simulink model "AdvancedMechM34"  (R2022b)
settings: Solver=FixedStepDiscrete  StartTime=0.0  StopTime=40  FixedStep=0.01  RelTol=1e-3  EnableMultiTasking=on
undefined symbols (not defined in the file): sigbuilder_block
settings Model: SILPILSystemUnderTest=refmodels  Creator=ahmed  LastModifiedBy=Mohamed
settings SolverCC: PositivePriorityOrder=on
settings OptimizationCC: EnhancedBackFolding=on  PassReuseOutputArgsAs=Individual arguments  ZeroExternalMemoryAtStartup=off  ZeroInternalMemoryAtStartup=off  MaxStackSize=64  OptimizeBlockOrder=speed  DifferentSizesBufferReuse=on  OptimizationCustomize=off  EfficientTunableParamExpr=on
settings DebuggingCC: ParameterTunabilityLossMsg=error
settings HardwareCC: ProdBitPerPointer=32  ProdBitPerSizeT=32  ProdBitPerPtrDiffT=32  ProdLargestAtomicInteger=Long  ProdLargestAtomicFloat=Double  ProdWordSize=32  ProdLongLongMode=on  ProdHWDeviceType=ARM Compatible->ARM Cortex
settings ModelReferenceCC: PropagateVarSize=During execution
settings RTWCC: Description=Embedded Coder  SystemTargetFile=ert.tlc  HardwareBoard=Raspberry Pi  TLCOptions="-aInlineSetEventsForThisBaseRateFcn=TLC_FALSE -aSuppressMultiTaskScheduler=TLC_FALSE  -aRateBasedStepFcn=0"  TemplateMakefile=ert_default_tmf  Toolchain=MinGW64 | gmake (64-bit Windows)  BuildConfiguration=Faster Runs
settings CodeAppCC: ForceParamTrailComments=on  IgnoreCustomStorageClasses=off  OperatorAnnotations=on  SimulinkDataObjDesc=on  SFDataObjDesc=on  InsertBlockDesc=on
settings ERTTargetCC: SupportContinuousTime=on  SupportVariableSizeSignals=on  ExtModeTransport=2  ExtModeStaticAlloc=on  ExtModeMexFile=ext_xcp  ExtModeIntrfLevel=Level2 - Open

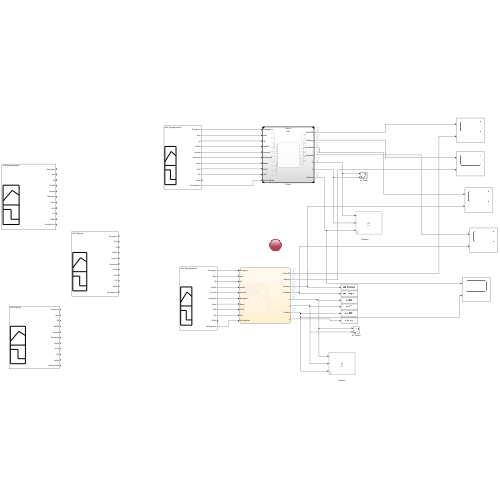
[thumbnail: Simulink's stored preview of the top-level diagram]
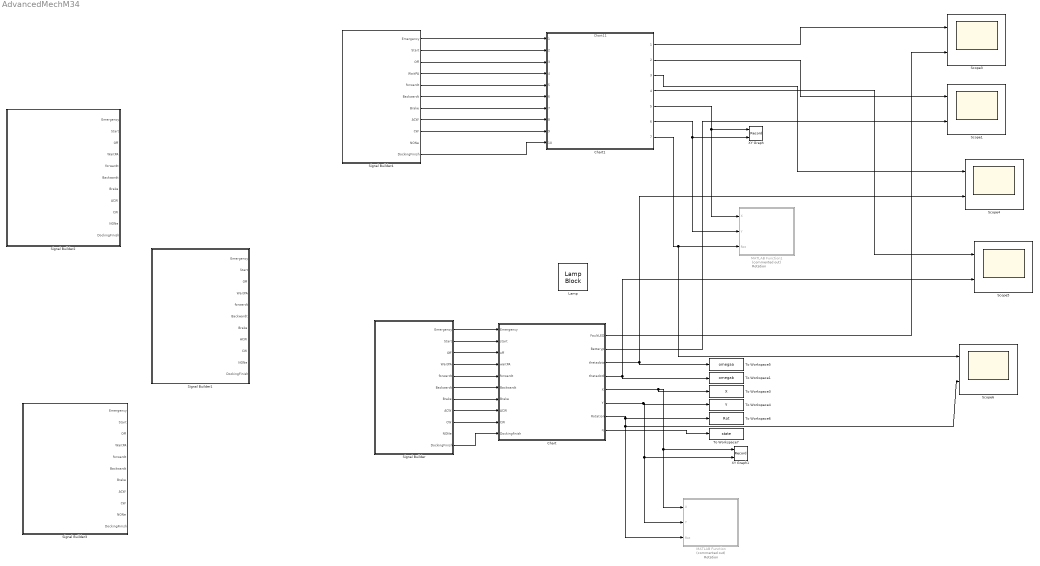
== system AdvancedMechM34 ==
  note: Rotation
  note: Rotation
  Chart : Stateflow chart  TreatAsAtomicUnit=on
  Chart1 : ModelReference  ModelNameDialog=Chart11  SimulationMode=Processor-in-the-loop (PIL)  ModelReferenceVersion=1.22
  Lamp : LampBlock  LabelPosition=Hide
  MATLAB Function : MATLAB Function  Commented=on  TreatAsAtomicUnit=on
  MATLAB Function1 : MATLAB Function  Commented=on  TreatAsAtomicUnit=on
  Scope{1,3..6} (5 alike) : Scope  NumInputPorts=2
  Signal Builder : Subsystem  Tag=STV Subsys  LoadFcn=sigbuilder_block('load');  StartFcn=sigbuilder_block('start');  StopFcn=sigbuilder_block('stop');  ClipboardFcn=sigbuilder_block('clipboard');  mask(Sigbuilder block){tuvar=[0:10]}
      mask help: Simulink:masks:SigbuilderBlock_MD
      mask init:
      | if ~strcmp(get_param(bdroot(gcbh),'SimulationStatus'),'stopped') tuvar = sigbuilder_block('maskInit'); end
      settings: CopyFcn=sigbuilder_block('copy');  DeleteFcn=sigbuilder_block('delete');  ModelCloseFcn=sigbuilder_block('modelClose');  PreSaveFcn=sigbuilder_block('preSave');  PauseFcn=sigbuilder_block('pause');  ContinueFcn=sigbuilder_block('continue');  NameChangeFcn=sigbuilder_block('namechange');  OpenFcn=sigbuilder_block('open',[5.4 5.4 1141.2 580.8 ]);  CloseFcn=sigbuilder_block('close');
      mask Display: plot(0, 0, 100, 100,[2, 2, 32, 32, 2], [68, 8, 8, 68, 68],[32, 2], [38, 38], [32, 19, 2],[53, 60, 44], [32, 17, 17, 2],[16, 16, 31, 31]);txt = getActiveGroup(gcbh);text(2, 100, txt,'verticalAlignment', 'top');
  Signal Builder1 : Subsystem  Tag=STV Subsys  LoadFcn=sigbuilder_block('load');  StartFcn=sigbuilder_block('start');  StopFcn=sigbuilder_block('stop');  ClipboardFcn=sigbuilder_block('clipboard');  mask(Sigbuilder block){tuvar=[0:10]}
      mask help: Simulink:masks:SigbuilderBlock_MD
      mask init:
      | if ~strcmp(get_param(bdroot(gcbh),'SimulationStatus'),'stopped') tuvar = sigbuilder_block('maskInit'); end
      settings: CopyFcn=sigbuilder_block('copy');  DeleteFcn=sigbuilder_block('delete');  ModelCloseFcn=sigbuilder_block('modelClose');  PreSaveFcn=sigbuilder_block('preSave');  PauseFcn=sigbuilder_block('pause');  ContinueFcn=sigbuilder_block('continue');  NameChangeFcn=sigbuilder_block('namechange');  OpenFcn=sigbuilder_block('open',[5.4 30 1141.2 522.6 ]);  CloseFcn=sigbuilder_block('close');
      mask Display: plot(0, 0, 100, 100,[2, 2, 32, 32, 2], [68, 8, 8, 68, 68],[32, 2], [38, 38], [32, 19, 2],[53, 60, 44], [32, 17, 17, 2],[16, 16, 31, 31]);txt = getActiveGroup(gcbh);text(2, 100, txt,'verticalAlignment', 'top');
  Signal Builder2 : Subsystem  Tag=STV Subsys  LoadFcn=sigbuilder_block('load');  StartFcn=sigbuilder_block('start');  StopFcn=sigbuilder_block('stop');  ClipboardFcn=sigbuilder_block('clipboard');  mask(Sigbuilder block){tuvar=[0:10]}
      mask help: Simulink:masks:SigbuilderBlock_MD
      mask init:
      | if ~strcmp(get_param(bdroot(gcbh),'SimulationStatus'),'stopped') tuvar = sigbuilder_block('maskInit'); end
      settings: CopyFcn=sigbuilder_block('copy');  DeleteFcn=sigbuilder_block('delete');  ModelCloseFcn=sigbuilder_block('modelClose');  PreSaveFcn=sigbuilder_block('preSave');  PauseFcn=sigbuilder_block('pause');  ContinueFcn=sigbuilder_block('continue');  NameChangeFcn=sigbuilder_block('namechange');  OpenFcn=sigbuilder_block('open',[5.4 5.4 1141.2 580.8 ]);  CloseFcn=sigbuilder_block('close');
      mask Display: plot(0, 0, 100, 100,[2, 2, 32, 32, 2], [68, 8, 8, 68, 68],[32, 2], [38, 38], [32, 19, 2],[53, 60, 44], [32, 17, 17, 2],[16, 16, 31, 31]);txt = getActiveGroup(gcbh);text(2, 100, txt,'verticalAlignment', 'top');
  Signal Builder3 : Subsystem  Tag=STV Subsys  LoadFcn=sigbuilder_block('load');  StartFcn=sigbuilder_block('start');  StopFcn=sigbuilder_block('stop');  ClipboardFcn=sigbuilder_block('clipboard');  mask(Sigbuilder block){tuvar=[0:10]}
      mask help: Simulink:masks:SigbuilderBlock_MD
      mask init:
      | if ~strcmp(get_param(bdroot(gcbh),'SimulationStatus'),'stopped') tuvar = sigbuilder_block('maskInit'); end
      settings: CopyFcn=sigbuilder_block('copy');  DeleteFcn=sigbuilder_block('delete');  ModelCloseFcn=sigbuilder_block('modelClose');  PreSaveFcn=sigbuilder_block('preSave');  PauseFcn=sigbuilder_block('pause');  ContinueFcn=sigbuilder_block('continue');  NameChangeFcn=sigbuilder_block('namechange');  OpenFcn=sigbuilder_block('open',[5.4 30 1141.2 522.6 ]);  CloseFcn=sigbuilder_block('close');
      mask Display: plot(0, 0, 100, 100,[2, 2, 32, 32, 2], [68, 8, 8, 68, 68],[32, 2], [38, 38], [32, 19, 2],[53, 60, 44], [32, 17, 17, 2],[16, 16, 31, 31]);txt = getActiveGroup(gcbh);text(2, 100, txt,'verticalAlignment', 'top');
  Signal Builder4 : Subsystem  Tag=STV Subsys  LoadFcn=sigbuilder_block('load');  StartFcn=sigbuilder_block('start');  StopFcn=sigbuilder_block('stop');  ClipboardFcn=sigbuilder_block('clipboard');  mask(Sigbuilder block){tuvar=[0:10]}
      mask help: Simulink:masks:SigbuilderBlock_MD
      mask init:
      | if ~strcmp(get_param(bdroot(gcbh),'SimulationStatus'),'stopped') tuvar = sigbuilder_block('maskInit'); end
      settings: CopyFcn=sigbuilder_block('copy');  DeleteFcn=sigbuilder_block('delete');  ModelCloseFcn=sigbuilder_block('modelClose');  PreSaveFcn=sigbuilder_block('preSave');  PauseFcn=sigbuilder_block('pause');  ContinueFcn=sigbuilder_block('continue');  NameChangeFcn=sigbuilder_block('namechange');  OpenFcn=sigbuilder_block('open',[5.4 5.4 1141.2 580.8 ]);  CloseFcn=sigbuilder_block('close');
      mask Display: plot(0, 0, 100, 100,[2, 2, 32, 32, 2], [68, 8, 8, 68, 68],[32, 2], [38, 38], [32, 19, 2],[53, 60, 44], [32, 17, 17, 2],[16, 16, 31, 31]);txt = getActiveGroup(gcbh);text(2, 100, txt,'verticalAlignment', 'top');
  To Workspace1 : ToWorkspace  VariableName=omegab  SampleTime=-1
  To Workspace3 : ToWorkspace  VariableName=X  SampleTime=-1
  To Workspace4 : ToWorkspace  VariableName=Y  SampleTime=-1
  To Workspace5 : ToWorkspace  VariableName=omegaa  SampleTime=-1
  To Workspace6 : ToWorkspace  VariableName=Rot  SampleTime=-1
  To Workspace7 : ToWorkspace  VariableName=state  SampleTime=-1
  XY Graph : Record  FileSettingsInternal="{\"entries\":[{\"content\":{\"excelSettings\":{\"content\":{},\"type\":\"Streamout.ExcelSettings\"}},\"type\":\"Streamout.FileSettingStorage\",\"uuid\":\"2d2e9be2-962d-486b-89bb-0fcf6ee4464c\"}],\"packageUris\":[\"http://schema.mathworks.com/mf0/streamout_blocks/R2020a\"],\"version\":\"1.0\"}"  Layout=[1 1]  SignalsInternal="{\"entries\":[{\"content\":{\"signals\":[{\"content\":{\"blockPath\":[\"AdvancedMechM34/XY Graph\"],\"channel\":[],\"dimensions\":[1],\"domain\":\"AdvancedMechM34/XY Graph\",\"lineColor\":\"#22b573\",\"plots\":[],\"port\":1,\"sid\":[\"\"],\"signalID\":9743,\"signalName\":\"Chart1:5\"},\"type\":\"RecordBlkView.Signal\",\"uuid\":\"d9327f8b-3fb2-4b96-8a94-861cd0cc077c\"},{\"content\":{\"blockPath\":[\"AdvancedMechM34/XY Graph\"],\"channel\":[],\"dimensions\":[1],\"domain\":\"AdvancedMechM34/XY Graph\",\"lineColor\":\"#0072bd\",\"plots\":[],\"port\":2,\"sid\":[\"\"],\"signalID\":9747,\"signalName\":\"Chart1:6\"},\"type\":\"RecordBlkView.Signal\",\"uuid\":\"b99db3ab-d58e-442b-9050-dd7db645c5da\"}]},\"type\":\"RecordBlkView.InputSignals\",\"uuid\":\"42776b80-9f46-428f-8740-cb522650dcbf\"}],\"packageUris\":[\"http://schema.mathworks.com/mf0/streamout_blocks/R2020a\"],\"version\":\"1.0\"}"  VisualizationBindings="{\"xyplotplugin\":{\"info\":[{\"series\":[],\"subplotID\":1}]}}"  CompatibilityTag=XY
  XY Graph1 : Record  FileSettingsInternal="{\"entries\":[{\"content\":{\"excelSettings\":{\"content\":{},\"type\":\"Streamout.ExcelSettings\"}},\"type\":\"Streamout.FileSettingStorage\",\"uuid\":\"0cb38b79-5d25-473b-896c-c2ddbf9cc01f\"}],\"packageUris\":[\"http://schema.mathworks.com/mf0/streamout_blocks/R2020a\"],\"version\":\"1.0\"}"  Layout=[1 1]  SignalsInternal="{\"entries\":[{\"content\":{\"signals\":[{\"content\":{\"blockPath\":[\"AdvancedMechM34/XY Graph1\"],\"channel\":[],\"dimensions\":[1],\"domain\":\"AdvancedMechM34/XY Graph1\",\"lineColor\":\"#7e2f8e\",\"plots\":[],\"port\":1,\"sid\":[\"\"],\"signalID\":9751,\"signalName\":\"Chart:5\"},\"type\":\"RecordBlkView.Signal\",\"uuid\":\"cda12369-6e26-4cba-9cb3-fbb7308e12dd\"},{\"content\":{\"blockPath\":[\"AdvancedMechM34/XY Graph1\"],\"channel\":[],\"dimensions\":[1],\"domain\":\"AdvancedMechM34/XY Graph1\",\"lineColor\":\"#77ac30\",\"plots\":[],\"port\":2,\"sid\":[\"\"],\"signalID\":9755,\"signalName\":\"Chart:6\"},\"type\":\"RecordBlkView.Signal\",\"uuid\":\"70410f22-8dbf-4caf-ba96-d8cd2bbc53f7\"}]},\"type\":\"RecordBlkView.InputSignals\",\"uuid\":\"4251f838-6728-4bbe-9a71-d6cba867fcff\"}],\"packageUris\":[\"http://schema.mathworks.com/mf0/streamout_blocks/R2020a\"],\"version\":\"1.0\"}"  VisualizationBindings="{\"xyplotplugin\":{\"info\":[{\"series\":[],\"subplotID\":1}]}}"  CompatibilityTag=XY
  wires:
  Chart/5(X) -> To Workspace3/1, XY Graph1/1, MATLAB Function/1(X)
  Chart/6(Y) -> To Workspace4/1, XY Graph1/2, MATLAB Function/2(Y)
  Chart/7(Rotation) -> To Workspace6/1, MATLAB Function/3(Rot), Scope6/2
  Chart1/6 -> MATLAB Function1/2(Y), XY Graph/2
  Chart1/7 -> Scope6/1, MATLAB Function1/3(Rot)
  Signal Builder4/1(Emergency) -> Chart1/1
  Signal Builder4/2(Start) -> Chart1/2
  Signal Builder4/3(Off) -> Chart1/3
  Signal Builder4/4(WaitPA) -> Chart1/4
  Signal Builder4/5(forwardt) -> Chart1/5
  Signal Builder4/6(Backwardt) -> Chart1/6
  Signal Builder4/7(Brake) -> Chart1/7
  Signal Builder4/8(ACW) -> Chart1/8
  Signal Builder4/9(CW) -> Chart1/9
  Signal Builder4/11(DockingFinish) -> Chart1/10
  Chart1/5 -> MATLAB Function1/1(X), XY Graph/1
  Signal Builder/1(Emergency) -> Chart/1(Emergency)
  Signal Builder/2(Start) -> Chart/2(start)
  Signal Builder/3(Off) -> Chart/3(off)
  Signal Builder/4(WaitPA) -> Chart/4(waitPA)
  Signal Builder/5(forwardt) -> Chart/5(forwardt)
  Signal Builder/6(Backwardt) -> Chart/6(Backwardt)
  Signal Builder/7(Brake) -> Chart/7(Brake)
  Signal Builder/8(ACW) -> Chart/8(ACW)
  Signal Builder/9(CW) -> Chart/9(CW)
  Signal Builder/11(DockingFinish) -> Chart/10(Dockingfinish)
  Chart1/1 -> Scope3/1
  Chart1/2 -> Scope1/1
  Chart1/3 -> Scope4/1
  Chart1/4 -> Scope5/1
  Chart/1(FaultLED) -> Scope3/2
  Chart/2(Batteryp) -> Scope1/2
  Chart/3(thetadota) -> Scope4/2, To Workspace5/1
  Chart/4(thetadotb) -> To Workspace1/1, Scope5/2
  Chart/8(q) -> To Workspace7/1

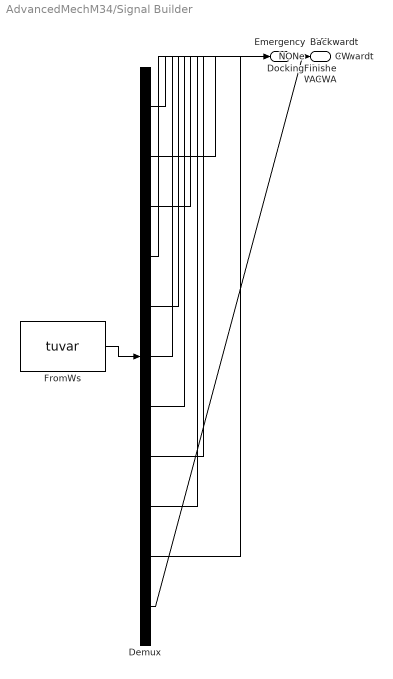
== system AdvancedMechM34/Signal Builder ==
  Demux : Demux  Tag=STV Demux  Outputs=11
      settings: DisplayOption=none
  FromWs : FromWorkspace  Tag=STV FromWs  VariableName=tuvar
      SigBuilderData=|
      | common.afterFinalStr = 'Extrapolate'
      | common.sampleTime = 0
      | dataSet.timeRange = [0 50]
      | dataSet.name = 'AGV SIgnals(case2)'
      | sbobj.Groups.Name = 'AGV SIgnals(case2)'
      | sbobj.Groups.Signals(1).Name = 'Emergency'
      | sbobj.Groups.Signals(1).XData = [0 4 6 7 7 10.45 10.45 50]
      | sbobj.Groups.Signals(1).YData = [0 0 0 0 1 1 0 0]
      | sbobj.Groups.Signals(2).Name = 'Start'
      | sbobj.Groups.Signals(2).XData = [0 0.99 1 1.5 1.5 9 9 11 11 14.1 14.1 16 16 50]
      | sbobj.Groups.Signals(2).YData = [0 0 1 1 0 0 1 1 0 0 1 1 0 0]
      | sbobj.Groups.Signals(3).Name = 'Off'
      | sbobj.Groups.Signals(3).XData = [0 11 50]
      | sbobj.Groups.Signals(3).YData = [0 0 0]
      | sbobj.Groups.Signals(4).Name = 'WaitPA'
      | sbobj.Groups.Signals(4).XData = [0 2.95 3.45 23 23 25 25 50]
      | sbobj.Groups.Signals(4).YData = [0 0 0 0 1 1 0 0]
      | sbobj.Groups.Signals(5).Name = 'forwardt'
      | sbobj.Groups.Signals(5).XData = [0 1.5 1.5 3 3.05 3.5 8 8 25.1 25.1 26.6 26.6 50]
      | sbobj.Groups.Signals(5).YData = [0 0 1 1 1 1 1 0 0 1 1 0 0]
      | sbobj.Groups.Signals(6).Name = 'Backwardt'
      | sbobj.Groups.Signals(6).XData = [0 50]
      | sbobj.Groups.Signals(6).YData = [0 0]
      | sbobj.Groups.Signals(7).Name = 'Brake'
      | sbobj.Groups.Signals(7).XData = [0 6.95 6.95 21 21 50]
      | sbobj.Groups.Signals(7).YData = [0 0 1 1 0 0]
      | sbobj.Groups.Signals(8).Name = 'ACW'
      | sbobj.Groups.Signals(8).XData = [0 50]
      | sbobj.Groups.Signals(8).YData = [0 0]
      | sbobj.Groups.Signals(9).Name = 'CW'
      | sbobj.Groups.Signals(9).XData = [0 50]
      | sbobj.Groups.Signals(9).YData = [0 0]
      | sbobj.Groups.Signals(10).Name = 'NONe'
      | sbobj.Groups.Signals(10).XData = [0 1.5 4 50]
      | sbobj.Groups.Signals(10).YData = [0 0 0 0]
      | sbobj.Groups.Signals(11).Name = 'DockingFinish'
      | sbobj.Groups.Signals(11).XData = [0 20.1 20.1 21.6 21.6 50]
      | sbobj.Groups.Signals(11).YData = [0 0 1 1 0 0]
      | sbobj.Groups.TimeRange = [0 50]
  Emergency : Outport  Tag=STV Outport
  Start : Outport  Tag=STV Outport  Port=2
  Off : Outport  Tag=STV Outport  Port=3
  WaitPA : Outport  Tag=STV Outport  Port=4
  forwardt : Outport  Tag=STV Outport  Port=5
  Backwardt : Outport  Tag=STV Outport  Port=6
  Brake : Outport  Tag=STV Outport  Port=7
  ACW : Outport  Tag=STV Outport  Port=8
  CW : Outport  Tag=STV Outport  Port=9
  NONe : Outport  Tag=STV Outport  Port=10
  DockingFinish : Outport  Tag=STV Outport  Port=11
  wires:
  Demux/1 -> Emergency/1
  FromWs/1 -> Demux/1
  Demux/2 -> Start/1
  Demux/3 -> Off/1
  Demux/4 -> WaitPA/1
  Demux/5 -> forwardt/1
  Demux/6 -> Backwardt/1
  Demux/7 -> Brake/1
  Demux/8 -> ACW/1
  Demux/9 -> CW/1
  Demux/10 -> NONe/1
  Demux/11 -> DockingFinish/1

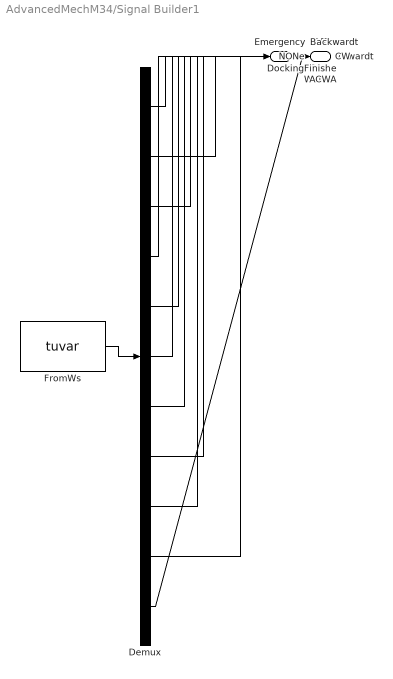
== system AdvancedMechM34/Signal Builder1 ==
  Demux : Demux  Tag=STV Demux  Outputs=11
      settings: DisplayOption=none
  FromWs : FromWorkspace  Tag=STV FromWs  VariableName=tuvar
      SigBuilderData=|
      | common.afterFinalStr = 'Extrapolate'
      | common.sampleTime = 0
      | dataSet.timeRange = [0 50]
      | dataSet.name = 'AGV SIgnals'
      | sbobj.Groups.Name = 'AGV SIgnals'
      | sbobj.Groups.Signals(1).Name = 'Emergency'
      | sbobj.Groups.Signals(1).XData = [0 4 6 7 7 9 9 50]
      | sbobj.Groups.Signals(1).YData = [0 0 0 0 1 1 0 0]
      | sbobj.Groups.Signals(2).Name = 'Start'
      | sbobj.Groups.Signals(2).XData = [0 0.99 1 1.5 1.5 9 9 11 11 14.1 14.1 16 16 50]
      | sbobj.Groups.Signals(2).YData = [0 0 1 1 0 0 1 1 0 0 1 1 0 0]
      | sbobj.Groups.Signals(3).Name = 'Off'
      | sbobj.Groups.Signals(3).XData = [0 11 11 14 14 30 30 50]
      | sbobj.Groups.Signals(3).YData = [0 0 1 1 0 0 1 1]
      | sbobj.Groups.Signals(4).Name = 'WaitPA'
      | sbobj.Groups.Signals(4).XData = [0 2.95 3.45 23 23 25 25 50]
      | sbobj.Groups.Signals(4).YData = [0 0 0 0 1 1 0 0]
      | sbobj.Groups.Signals(5).Name = 'forwardt'
      | sbobj.Groups.Signals(5).XData = [0 1.5 1.5 3 3.05 3.5 8 8 25.1 25.1 26.6 26.6 50]
      | sbobj.Groups.Signals(5).YData = [0 0 1 1 1 1 1 0 0 1 1 0 0]
      | sbobj.Groups.Signals(6).Name = 'Backwardt'
      | sbobj.Groups.Signals(6).XData = [0 16 16 17 17 50]
      | sbobj.Groups.Signals(6).YData = [0 0 1 1 0 0]
      | sbobj.Groups.Signals(7).Name = 'Brake'
      | sbobj.Groups.Signals(7).XData = [0 20 20 21 21 50]
      | sbobj.Groups.Signals(7).YData = [0 0 1 1 0 0]
      | sbobj.Groups.Signals(8).Name = 'ACW'
      | sbobj.Groups.Signals(8).XData = [0 5 5 5.5 8.55 17 18 18 50]
      | sbobj.Groups.Signals(8).YData = [0 0 1 1 1 1 1 0 0]
      | sbobj.Groups.Signals(9).Name = 'CW'
      | sbobj.Groups.Signals(9).XData = [0 2.6 2.6 4.1 5 5 50]
      | sbobj.Groups.Signals(9).YData = [0 0 1 1 1 0 0]
      | sbobj.Groups.Signals(10).Name = 'NONe'
      | sbobj.Groups.Signals(10).XData = [0 1.5 4 50]
      | sbobj.Groups.Signals(10).YData = [0 0 0 0]
      | sbobj.Groups.Signals(11).Name = 'DockingFinish'
      | sbobj.Groups.Signals(11).XData = [0 20.1 20.1 21.6 21.6 50]
      | sbobj.Groups.Signals(11).YData = [0 0 1 1 0 0]
      | sbobj.Groups.TimeRange = [0 50]
  Emergency : Outport  Tag=STV Outport
  Start : Outport  Tag=STV Outport  Port=2
  Off : Outport  Tag=STV Outport  Port=3
  WaitPA : Outport  Tag=STV Outport  Port=4
  forwardt : Outport  Tag=STV Outport  Port=5
  Backwardt : Outport  Tag=STV Outport  Port=6
  Brake : Outport  Tag=STV Outport  Port=7
  ACW : Outport  Tag=STV Outport  Port=8
  CW : Outport  Tag=STV Outport  Port=9
  NONe : Outport  Tag=STV Outport  Port=10
  DockingFinish : Outport  Tag=STV Outport  Port=11
  wires:
  Demux/1 -> Emergency/1
  FromWs/1 -> Demux/1
  Demux/2 -> Start/1
  Demux/3 -> Off/1
  Demux/4 -> WaitPA/1
  Demux/5 -> forwardt/1
  Demux/6 -> Backwardt/1
  Demux/7 -> Brake/1
  Demux/8 -> ACW/1
  Demux/9 -> CW/1
  Demux/10 -> NONe/1
  Demux/11 -> DockingFinish/1

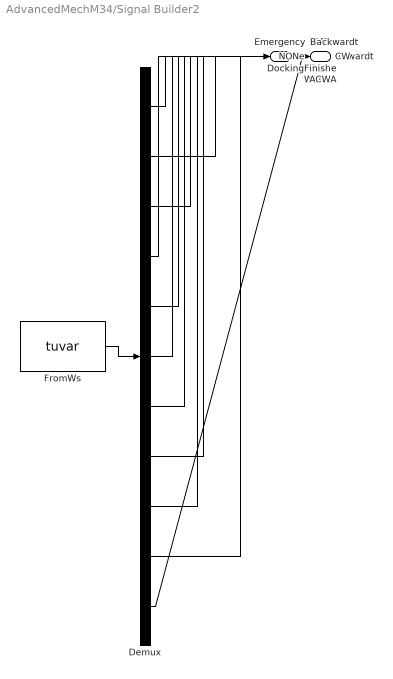
== system AdvancedMechM34/Signal Builder2 ==
  Demux : Demux  Tag=STV Demux  Outputs=11
      settings: DisplayOption=none
  FromWs : FromWorkspace  Tag=STV FromWs  VariableName=tuvar
      SigBuilderData=|
      | common.afterFinalStr = 'Extrapolate'
      | common.sampleTime = 0
      | dataSet.timeRange = [0 50]
      | dataSet.name = 'AGV SIgnals(case3)'
      | sbobj.Groups.Name = 'AGV SIgnals(case3)'
      | sbobj.Groups.Signals(1).Name = 'Emergency'
      | sbobj.Groups.Signals(1).XData = [0 4 6 7 10.45 50]
      | sbobj.Groups.Signals(1).YData = [0 0 0 0 0 0]
      | sbobj.Groups.Signals(2).Name = 'Start'
      | sbobj.Groups.Signals(2).XData = [0 0.1 1.5 1.5 9 11 14.1 50]
      | sbobj.Groups.Signals(2).YData = [0 1 1 0 0 0 0 0]
      | sbobj.Groups.Signals(3).Name = 'Off'
      | sbobj.Groups.Signals(3).XData = [0 11 50]
      | sbobj.Groups.Signals(3).YData = [0 0 0]
      | sbobj.Groups.Signals(4).Name = 'WaitPA'
      | sbobj.Groups.Signals(4).XData = [0 2.95 3.45 30.9 30.9 34.7 34.7 50]
      | sbobj.Groups.Signals(4).YData = [0 0 0 0 1 1 0 0]
      | sbobj.Groups.Signals(5).Name = 'forwardt'
      | sbobj.Groups.Signals(5).XData = [0 0.35 0.35 3 3.05 3.5 15.1 15.1 25.1 25.1 26.6 26.6 50]
      | sbobj.Groups.Signals(5).YData = [0 0 1 1 1 1 1 0 0 1 1 0 0]
      | sbobj.Groups.Signals(6).Name = 'Backwardt'
      | sbobj.Groups.Signals(6).XData = [0 50]
      | sbobj.Groups.Signals(6).YData = [0 0]
      | sbobj.Groups.Signals(7).Name = 'Brake'
      | sbobj.Groups.Signals(7).XData = [0 36.7 36.7 43.3 43.3 50]
      | sbobj.Groups.Signals(7).YData = [0 0 1 1 0 0]
      | sbobj.Groups.Signals(8).Name = 'ACW'
      | sbobj.Groups.Signals(8).XData = [0 50]
      | sbobj.Groups.Signals(8).YData = [0 0]
      | sbobj.Groups.Signals(9).Name = 'CW'
      | sbobj.Groups.Signals(9).XData = [0 5.95 5.95 34.9 34.9 50]
      | sbobj.Groups.Signals(9).YData = [0 0 1 1 0 0]
      | sbobj.Groups.Signals(10).Name = 'NONe'
      | sbobj.Groups.Signals(10).XData = [0 1.5 4 50]
      | sbobj.Groups.Signals(10).YData = [0 0 0 0]
      | sbobj.Groups.Signals(11).Name = 'DockingFinish'
      | sbobj.Groups.Signals(11).XData = [0 20.1 20.1 21.6 21.6 50]
      | sbobj.Groups.Signals(11).YData = [0 0 1 1 0 0]
      | sbobj.Groups.TimeRange = [0 50]
  Emergency : Outport  Tag=STV Outport
  Start : Outport  Tag=STV Outport  Port=2
  Off : Outport  Tag=STV Outport  Port=3
  WaitPA : Outport  Tag=STV Outport  Port=4
  forwardt : Outport  Tag=STV Outport  Port=5
  Backwardt : Outport  Tag=STV Outport  Port=6
  Brake : Outport  Tag=STV Outport  Port=7
  ACW : Outport  Tag=STV Outport  Port=8
  CW : Outport  Tag=STV Outport  Port=9
  NONe : Outport  Tag=STV Outport  Port=10
  DockingFinish : Outport  Tag=STV Outport  Port=11
  wires:
  Demux/1 -> Emergency/1
  FromWs/1 -> Demux/1
  Demux/2 -> Start/1
  Demux/3 -> Off/1
  Demux/4 -> WaitPA/1
  Demux/5 -> forwardt/1
  Demux/6 -> Backwardt/1
  Demux/7 -> Brake/1
  Demux/8 -> ACW/1
  Demux/9 -> CW/1
  Demux/10 -> NONe/1
  Demux/11 -> DockingFinish/1

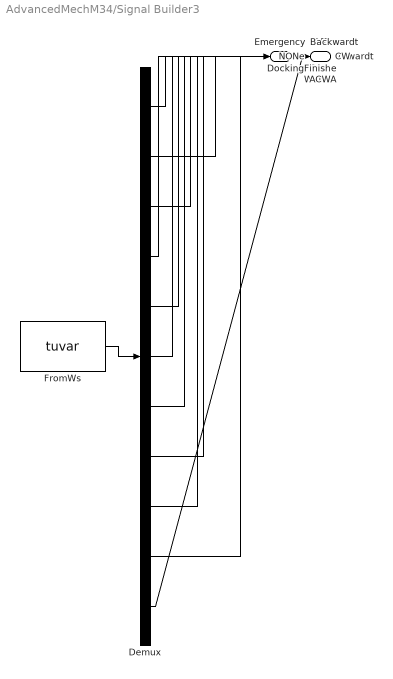
== system AdvancedMechM34/Signal Builder3 ==
  Demux : Demux  Tag=STV Demux  Outputs=11
      settings: DisplayOption=none
  FromWs : FromWorkspace  Tag=STV FromWs  VariableName=tuvar
      SigBuilderData=|
      | common.afterFinalStr = 'Extrapolate'
      | common.sampleTime = 0
      | dataSet.timeRange = [0 50]
      | dataSet.name = 'AGV SIgnals'
      | sbobj.Groups.Name = 'AGV SIgnals'
      | sbobj.Groups.Signals(1).Name = 'Emergency'
      | sbobj.Groups.Signals(1).XData = [0 4 6 7 7 9 9 50]
      | sbobj.Groups.Signals(1).YData = [0 0 0 0 1 1 0 0]
      | sbobj.Groups.Signals(2).Name = 'Start'
      | sbobj.Groups.Signals(2).XData = [0 0.99 1 1.5 1.5 9 9 11 11 14.1 16 50]
      | sbobj.Groups.Signals(2).YData = [0 0 1 1 0 0 1 1 0 0 0 0]
      | sbobj.Groups.Signals(3).Name = 'Off'
      | sbobj.Groups.Signals(3).XData = [0 11 14 30 30 50]
      | sbobj.Groups.Signals(3).YData = [0 0 0 0 1 1]
      | sbobj.Groups.Signals(4).Name = 'WaitPA'
      | sbobj.Groups.Signals(4).XData = [0 2.95 3.45 23 23 25 25 50]
      | sbobj.Groups.Signals(4).YData = [0 0 0 0 1 1 0 0]
      | sbobj.Groups.Signals(5).Name = 'forwardt'
      | sbobj.Groups.Signals(5).XData = [0 1.5 1.5 3 3.05 3.5 8 8 25.1 25.1 26.6 26.6 50]
      | sbobj.Groups.Signals(5).YData = [0 0 1 1 1 1 1 0 0 1 1 0 0]
      | sbobj.Groups.Signals(6).Name = 'Backwardt'
      | sbobj.Groups.Signals(6).XData = [0 11.6 11.6 13.5 13.5 16 16 17 17 50]
      | sbobj.Groups.Signals(6).YData = [0 0 1 1 0 0 1 1 0 0]
      | sbobj.Groups.Signals(7).Name = 'Brake'
      | sbobj.Groups.Signals(7).XData = [0 20 20 21 21 50]
      | sbobj.Groups.Signals(7).YData = [0 0 1 1 0 0]
      | sbobj.Groups.Signals(8).Name = 'ACW'
      | sbobj.Groups.Signals(8).XData = [0 5 5 5.5 8.55 17 18 18 50]
      | sbobj.Groups.Signals(8).YData = [0 0 1 1 1 1 1 0 0]
      | sbobj.Groups.Signals(9).Name = 'CW'
      | sbobj.Groups.Signals(9).XData = [0 2.6 2.6 4.1 5 5 50]
      | sbobj.Groups.Signals(9).YData = [0 0 1 1 1 0 0]
      | sbobj.Groups.Signals(10).Name = 'NONe'
      | sbobj.Groups.Signals(10).XData = [0 1.5 4 50]
      | sbobj.Groups.Signals(10).YData = [0 0 0 0]
      | sbobj.Groups.Signals(11).Name = 'DockingFinish'
      | sbobj.Groups.Signals(11).XData = [0 20.1 20.1 21.6 21.6 50]
      | sbobj.Groups.Signals(11).YData = [0 0 1 1 0 0]
      | sbobj.Groups.TimeRange = [0 50]
  Emergency : Outport  Tag=STV Outport
  Start : Outport  Tag=STV Outport  Port=2
  Off : Outport  Tag=STV Outport  Port=3
  WaitPA : Outport  Tag=STV Outport  Port=4
  forwardt : Outport  Tag=STV Outport  Port=5
  Backwardt : Outport  Tag=STV Outport  Port=6
  Brake : Outport  Tag=STV Outport  Port=7
  ACW : Outport  Tag=STV Outport  Port=8
  CW : Outport  Tag=STV Outport  Port=9
  NONe : Outport  Tag=STV Outport  Port=10
  DockingFinish : Outport  Tag=STV Outport  Port=11
  wires:
  Demux/1 -> Emergency/1
  FromWs/1 -> Demux/1
  Demux/2 -> Start/1
  Demux/3 -> Off/1
  Demux/4 -> WaitPA/1
  Demux/5 -> forwardt/1
  Demux/6 -> Backwardt/1
  Demux/7 -> Brake/1
  Demux/8 -> ACW/1
  Demux/9 -> CW/1
  Demux/10 -> NONe/1
  Demux/11 -> DockingFinish/1

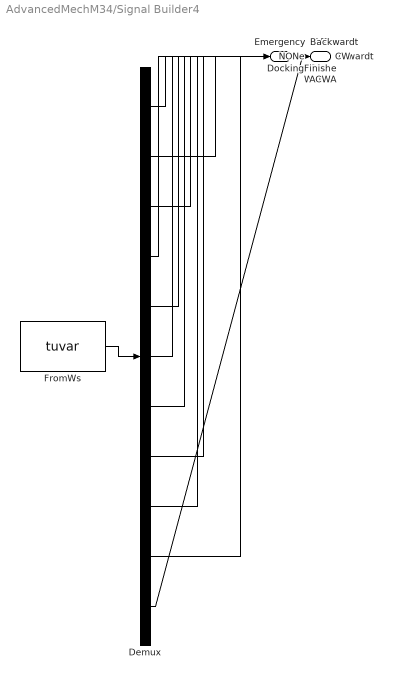
== system AdvancedMechM34/Signal Builder4 ==
  Demux : Demux  Tag=STV Demux  Outputs=11
      settings: DisplayOption=none
  FromWs : FromWorkspace  Tag=STV FromWs  VariableName=tuvar
      SigBuilderData=|
      | common.afterFinalStr = 'Extrapolate'
      | common.sampleTime = 0
      | dataSet.timeRange = [0 50]
      | dataSet.name = 'AGV SIgnals(case2)'
      | sbobj.Groups.Name = 'AGV SIgnals(case2)'
      | sbobj.Groups.Signals(1).Name = 'Emergency'
      | sbobj.Groups.Signals(1).XData = [0 4 6 7 7 10.45 10.45 50]
      | sbobj.Groups.Signals(1).YData = [0 0 0 0 1 1 0 0]
      | sbobj.Groups.Signals(2).Name = 'Start'
      | sbobj.Groups.Signals(2).XData = [0 0.99 1 1.5 1.5 9 9 11 11 14.1 14.1 16 16 50]
      | sbobj.Groups.Signals(2).YData = [0 0 1 1 0 0 1 1 0 0 1 1 0 0]
      | sbobj.Groups.Signals(3).Name = 'Off'
      | sbobj.Groups.Signals(3).XData = [0 11 50]
      | sbobj.Groups.Signals(3).YData = [0 0 0]
      | sbobj.Groups.Signals(4).Name = 'WaitPA'
      | sbobj.Groups.Signals(4).XData = [0 2.95 3.45 23 23 25 25 50]
      | sbobj.Groups.Signals(4).YData = [0 0 0 0 1 1 0 0]
      | sbobj.Groups.Signals(5).Name = 'forwardt'
      | sbobj.Groups.Signals(5).XData = [0 1.5 1.5 3 3.05 3.5 8 8 25.1 25.1 26.6 26.6 50]
      | sbobj.Groups.Signals(5).YData = [0 0 1 1 1 1 1 0 0 1 1 0 0]
      | sbobj.Groups.Signals(6).Name = 'Backwardt'
      | sbobj.Groups.Signals(6).XData = [0 50]
      | sbobj.Groups.Signals(6).YData = [0 0]
      | sbobj.Groups.Signals(7).Name = 'Brake'
      | sbobj.Groups.Signals(7).XData = [0 6.95 6.95 21 21 50]
      | sbobj.Groups.Signals(7).YData = [0 0 1 1 0 0]
      | sbobj.Groups.Signals(8).Name = 'ACW'
      | sbobj.Groups.Signals(8).XData = [0 50]
      | sbobj.Groups.Signals(8).YData = [0 0]
      | sbobj.Groups.Signals(9).Name = 'CW'
      | sbobj.Groups.Signals(9).XData = [0 50]
      | sbobj.Groups.Signals(9).YData = [0 0]
      | sbobj.Groups.Signals(10).Name = 'NONe'
      | sbobj.Groups.Signals(10).XData = [0 1.5 4 50]
      | sbobj.Groups.Signals(10).YData = [0 0 0 0]
      | sbobj.Groups.Signals(11).Name = 'DockingFinish'
      | sbobj.Groups.Signals(11).XData = [0 20.1 20.1 21.6 21.6 50]
      | sbobj.Groups.Signals(11).YData = [0 0 1 1 0 0]
      | sbobj.Groups.TimeRange = [0 50]
  Emergency : Outport  Tag=STV Outport
  Start : Outport  Tag=STV Outport  Port=2
  Off : Outport  Tag=STV Outport  Port=3
  WaitPA : Outport  Tag=STV Outport  Port=4
  forwardt : Outport  Tag=STV Outport  Port=5
  Backwardt : Outport  Tag=STV Outport  Port=6
  Brake : Outport  Tag=STV Outport  Port=7
  ACW : Outport  Tag=STV Outport  Port=8
  CW : Outport  Tag=STV Outport  Port=9
  NONe : Outport  Tag=STV Outport  Port=10
  DockingFinish : Outport  Tag=STV Outport  Port=11
  wires:
  Demux/1 -> Emergency/1
  FromWs/1 -> Demux/1
  Demux/2 -> Start/1
  Demux/3 -> Off/1
  Demux/4 -> WaitPA/1
  Demux/5 -> forwardt/1
  Demux/6 -> Backwardt/1
  Demux/7 -> Brake/1
  Demux/8 -> ACW/1
  Demux/9 -> CW/1
  Demux/10 -> NONe/1
  Demux/11 -> DockingFinish/1

== matlab function AdvancedMechM34/MATLAB Function ==
  data: X input; Y input; Rot input
function fcn(X,Y,Rot)
radius =1;
plot(0);
hold on
xlim([X-5,X+5]); %define limits in X-direction
ylim([Y-5,Y+5]); %define limits in Y-direction
grid on; %initialize the grid to be on
axis square; %make the axes look like square
th = 0:pi/50:2*pi;
xunit = radius * cos(th) + X;
yunit = radius * sin(th) + Y;
    plot(xunit, yunit);
    plot(X+radius*cos(Rot), Y+radius*sin(Rot), 'Kx');
drawnow;   
hold off

== stateflow chart AdvancedMechM34/Chart ==
  state ON
    state Active_task [parallel]
      during:
      q=q1*10+q2;
      exit:
      q=00;
      settings: executionOrder=1
      state Motion
        state Translational [parallel]
          exit:
          t=0;
          settings: executionOrder=1
          state Forward
            entry:
            q1=1
            t=1
          state Backward
            entry:
            q1=2
            t=-1
          state none
            entry:
            q1=0
            t=0
          ON.Active_task.Motion.Translational.none -> Forward [order 2] : [forwardt==1]
          Forward -> ON.Active_task.Motion.Translational.none [order 1] : [Brake==1]
          Forward -> Backward [order 2] : [Backwardt==1]
          Backward -> Forward [order 1] : [forwardt==1]
          ON.Active_task.Motion.Translational.none -> Backward [order 1] : [Backwardt==1]
          Backward -> ON.Active_task.Motion.Translational.none [order 2] : [Brake==1]
          (default) -> ON.Active_task.Motion.Translational.none
          ON.Active_task.Motion.Translational.none -> ON.Active_task.Motion.Translational.none [order 3] : [Brake==1]
        state Rotational [parallel]
          exit:
          r=0;
          settings: executionOrder=2
          state CLCK_WISE
            entry:
            q2=1;
            r=-1
          state Anti_CLCKWISE
            entry:
            q2=2
            r=1
          state none
            entry:
            q2=0;
            r=0
          ON.Active_task.Motion.Rotational.none -> CLCK_WISE [order 2] : [CW==1]
          CLCK_WISE -> ON.Active_task.Motion.Rotational.none [order 2] : [Brake==1]
          Anti_CLCKWISE -> CLCK_WISE [order 2] : [CW==1]
          CLCK_WISE -> Anti_CLCKWISE [order 1] : [ACW==1]
          ON.Active_task.Motion.Rotational.none -> Anti_CLCKWISE [order 1] : [ACW==1]
          Anti_CLCKWISE -> ON.Active_task.Motion.Rotational.none [order 1] : [Brake==1]
          (default) -> ON.Active_task.Motion.Rotational.none
          ON.Active_task.Motion.Rotational.none -> ON.Active_task.Motion.Rotational.none [order 3] : [Brake==1]
      state Charging_station
        state Docking
          exit:
          d=1;
        state Docked
          exit:
          d=0;
        Docking -> Docked : [Dockingfinish==1]
        (default) -> Docking
      state Waiting
        entry:
        r=0;
        t=0;
        during:
        if ( forwardt || Backwardt || CW || ACW == 1)
        g=1;
        end
        exit:
        g=0;
      Motion -> Charging_station [order 2] : [Batteryp<=30]
      (default) -> Motion
      Charging_station -> Motion : [Batteryp==100]
      Waiting -> Motion : [g==1 & waitPA ==0]
      Motion -> Waiting [order 1] : [waitPA==1]
    state Continuous [parallel]
      entry:
      %setting DCmotor Conditions
      J=0.01;
      b=0.1;
      Ke=0.01;
      Kt=0.01;
      R=1;
      L=0.5;
      Ts = 0.01;
      %%setting AGV parameters
      radius = 1;
      wheelradius=0.1;
      during:
      %using t and r to find motor speeds
      Va_Desired = 5*(t + (0.4/2)* r);
      Vb_Desired=  5*(t - (0.4/2)* r);
      %First Motor Equations
      thetadoubledota = (1/J)*(Kt*ia-b*thetadota);
      idota = (1/L)*(-R*ia+input_MotorA-Ke*thetadota);
      ia=ia+idota*Ts;
      thetadota=thetadota+thetadoubledota*Ts;
      %%second Motor Equations
      thetadoubledotb = (1/J)*(Kt*ib-b*thetadotb);
      idotb = (1/L)*(-1*ib+input_MotorB-Ke*thetadotb);
      ib=ib+idotb*Ts;
      thetadotb=thetadotb+thetadoubledotb*Ts;
      %%updating Current taken from battery
      Id=ia+ib;
      %% Updating X Y and Rotation of AGV
      Va =  thetadota* wheelradius;
      Vb = thetadotb*wheelradius;
      Vt=(Va+Vb)/2;
      rotationSpeed=(Va-Vb)/radius;
      Rotation = Rotation+rotationSpeed*Ts;
      X=X+Vt*cos(Rotation)*Ts;
      Y=Y+Vt*sin(Rotation)*Ts;
      settings: executionOrder=3
    state Battery_management [parallel]
      settings: executionOrder=2
      state Charging
        during:
        SOC = SOC + I*Ts
        if(SOC>=100000)
        SOC=100000
        end
        Batteryp = (SOC/100000)*100
      state Discharging
        during:
        SOC = SOC - abs(Id)*Ts
        if(SOC>=100000)
        SOC=100000
        end
        Batteryp = (SOC/100000)*100
      (default) -> Discharging
      Charging -> Discharging : [d==0]
      Discharging -> Charging : [d==1]
    state PID_Controller [parallel]
      %% First Controller
      Kp=40;
      Ki=100;
      Kd=0.01;
      Error_old_MotorA= Error_MotorA;
      Error_MotorA =Va_Desired/wheelradius-thetadota;
      inte_MotorA = inte_MotorA+Error_MotorA*Ts;
      Diff_MotorA = (Error_MotorA-Error_old_MotorA)/Ts;
      input_MotorA = Kp*Error_MotorA+Ki*inte_MotorA+Kd*Diff_MotorA;
      %% Second Controller
      Kp=40;
      Ki=100;
      Kd=0.01;
      Error_old_MotorB= Error_MotorB;
      Error_MotorB =Vb_Desired/wheelradius-thetadotb;
      inte_MotorB = inte_MotorB+Error_MotorB*Ts;
      Diff_MotorB = (Error_MotorB-Error_old_MotorB)/Ts;
      input_MotorB = Kp*Error_MotorB+Ki*inte_MotorB+Kd*Diff_MotorB;
      settings: executionOrder=4
  state OFF
    entry:
    r=0
    t=0
    thetadota=0;
    thetadotb=0;
  state Emergency
    entry:
    FaultLED=1;
    r=0;
    t=0;
    thetadota=0;
    thetadotb=0;
    exit:
    FaultLED=0;
  Emergency -> ON : [start==1 && Emergency==0]
  ON -> Emergency [order 2] : [Emergency==1]
  (default) -> OFF
  OFF -> ON : [start==1]
  ON -> OFF [order 1] : [off==1]
  data: FaultLED output; Emergency input; start input; off input; waitPA input; forwardt input; Backwardt input; Brake input; ACW input; CW input; Batteryp output =100; I local =100; SOC local =100000; d local =0; Dockingfinish input; g local =0; t local; r local; Id local =0; J local =0; Ke local =0; Kt local =0; L local =0; R local =0; Ts local =0; Va local =0; Vb local =0; b local =0; ia local =0; ib local =0; idota local =0; idotb local =0; thetadoubledota local =0; thetadoubledotb local =0; thetadota output =0; thetadotb output =0; Diff_MotorA local =0; Diff_MotorB local =0; Error_MotorA local =0; Error_MotorB local =0; Error_old_MotorA local =0; Error_old_MotorB local =0; Kd local =0; Ki local =00; Kp local =00; input_MotorA local =0; input_MotorB local =0; inte_MotorA local =0; inte_MotorB local =0; radius local =0; Va_Desired local =0; Vb_Desired local =0; Vt local =0; rotationSpeed local =0; wheelradius local =0; X output =0; Y output =0; Rotation output =0; q output; q1 local; q2 local

== matlab function AdvancedMechM34/MATLAB Function1 ==
  data: X input; Y input; Rot input
function fcn(X,Y,Rot)
radius =1;
plot(0);
hold on
xlim([X-5,X+5]); %define limits in X-direction
ylim([Y-5,Y+5]); %define limits in Y-direction
grid on; %initialize the grid to be on
axis square; %make the axes look like square
th = 0:pi/50:2*pi;
xunit = radius * cos(th) + X;
yunit = radius * sin(th) + Y;
    plot(xunit, yunit);
    plot(X+radius*cos(Rot), Y+radius*sin(Rot), 'Kx');
drawnow;   
hold off
